simulink model "simuMotoreducteur"  (R2017a)
settings: Solver=VariableStepAuto  StartTime=0.0  StopTime=0.2  RelTol=1e-3
settings Model: Creator=Alex  LastModifiedBy=Alex
settings DataIOCC: ReturnWorkspaceOutputs=on
settings SFSimCC: SimUseLocalCustomCode=on
settings RTWCC: RTWUseLocalCustomCode=on

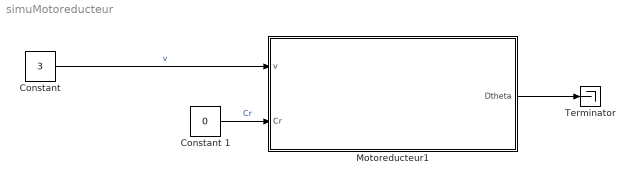
== system simuMotoreducteur ==
  "Constant " : Constant  Value=3
  Constant 1 : Constant  Value=0
  Motoreducteur1 : Subsystem  mask{L=1e-3, R=4.42, J=7.32e-4, k=0.4646, i0=0, Dtheta0=0}
      mask prompts: L "Electrical inductance"; R "Electrival resistance"; J "Inertia"; k "Electomechanical constant"; i0 "current"; Dtheta0 "speed"
  Terminator : Terminator
  wires:
  "Constant "/1 -> Motoreducteur1/1(v)  "v"
  Constant 1/1 -> Motoreducteur1/2(Cr)  "Cr"
  Motoreducteur1/1(Dtheta) -> Terminator/1

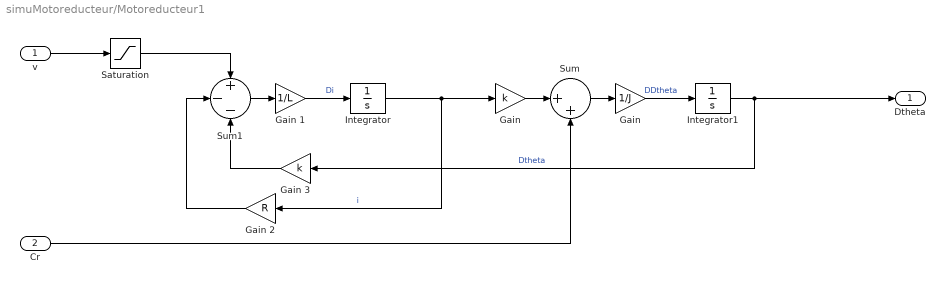
== system simuMotoreducteur/Motoreducteur1 ==
  v : Inport
  Cr : Inport  Port=2
  "Gain " : Gain  Gain=1/J
  "Gain  " : Gain  Gain=k
  Gain 1 : Gain  Gain=1/L
  Gain 2 : Gain  Gain=R
  Gain 3 : Gain  Gain=k
  Integrator : Integrator  InitialCondition=i0
  Integrator1 : Integrator  InitialCondition=Dtheta0
  Saturation : Saturate  UpperLimit=9  LowerLimit=-9
  Sum : Sum  Inputs=|++
  Sum1 : Sum  Inputs=+--
  Dtheta : Outport
  wires:
  Saturation/1 -> Sum1/1
  Gain 3/1 -> Sum1/3
  Integrator/1 -> "Gain  "/1, Gain 2/1  "i"
  Sum/1 -> "Gain "/1
  Cr/1 -> Sum/2
  Gain 1/1 -> Integrator/1  "Di"
  v/1 -> Saturation/1
  Sum1/1 -> Gain 1/1
  Integrator1/1 -> Gain 3/1, Dtheta/1  "Dtheta"
  Gain 2/1 -> Sum1/2
  "Gain "/1 -> Integrator1/1  "DDtheta"
  "Gain  "/1 -> Sum/1
